simulink model "prototype_multiple_msg"  (R2021b)
settings: Solver=FixedStepDiscrete  StartTime=0.0  StopTime=Inf  FixedStep=1  RelTol=1e-3
settings Model: Creator=vgaggero  LastModifiedBy=grodriguez
settings SolverCC: AllowMultiTaskInputOutput=on  AutoInsertRateTranBlk=on  InsertRTBMode=Never (minimum delay)

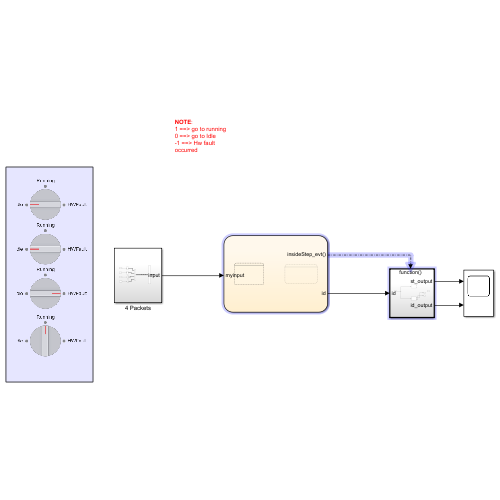
[thumbnail: Simulink's stored preview of the top-level diagram]
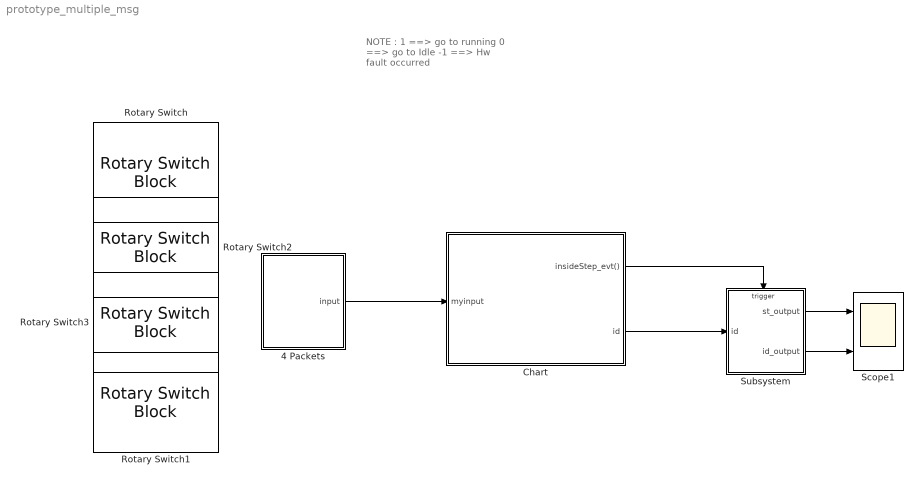
== system prototype_multiple_msg ==
  note: NOTE :
      | 1 ==> go to running
      | 0 ==> go to Idle
      | -1 ==> Hw fault occurred
  4 Packets : Subsystem
  Chart : Stateflow chart  TreatAsAtomicUnit=on
      settings: PortSchema="{\"entries\":[{\"content\":{\"sides\":[{\"content\":{\"connectorIds\":[\"In1\"]},\"type\":\"ConnectorPlacement.EquallySpacedRectSide\",\"uuid\":\"6cfd0d6c-bd6f-4458-8e18-10a89c7a7397\"},{\"content\":{\"connectorIds\":[\"Out2\",\"Out1\"],\"side\":\"RIGHT\"},\"type\":\"ConnectorPlacement.EquallySpacedRectSide\",\"uuid\":\"2cbad870-62d0-4bb8-9198-36e7d278500c\"},{\"content\":{\"connectorIds\":[],\"side\":\"TOP\"},\"type\":\"ConnectorPlacement.EquallySpacedRectSide\",\"uuid\":\"c9b4a32e-c2b5-43d7-b3cd-6996e0fae254\"}]},\"type\":\"ConnectorPlacement.EquallySpacedConnector\",\"uuid\":\"e32f82e2-d4b7-4dda-bf5a-9df2c9c9d870\"}],\"packageUris\":[\"http://schema.mathworks.com/mf0/Connector/R2020b\"],\"version\":\"1.0\"}"
  Rotary Switch{,1..3} (4 alike) : RotarySwitchBlock  LabelPosition=Hide
      settings: Values={{'Idle', 'Running', 'HWFault'}, [0 1 -1]}
  Scope1 : Scope  NumInputPorts=2
  Subsystem : Subsystem
  wires:
  Chart/2(insideStep_evt()) -> Subsystem/Trigger
  Chart/1(id) -> Subsystem/1(id)
  Subsystem/1(st_output) -> Scope1/1
  Subsystem/2(id_output) -> Scope1/2
  4 Packets/1(input) -> Chart/1(myinput)

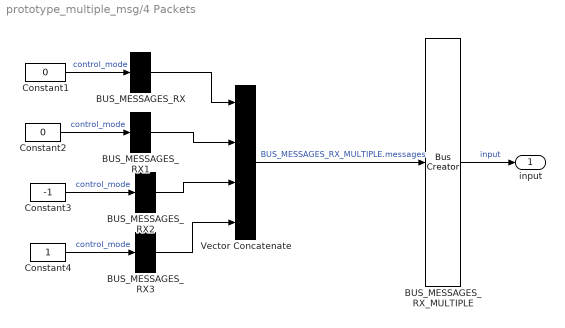
== system prototype_multiple_msg/4 Packets ==
  BUS_MESSAGES_RX{,1..3} (4 alike) : BusCreator  Inputs=1  OutDataTypeStr=Bus: BUS_MESSAGES_RX  NonVirtualBus=on
  BUS_MESSAGES_RX_MULTIPLE : BusCreator  Inputs=1  OutDataTypeStr=Bus: BUS_MESSAGES_RX_MULTIPLE  NonVirtualBus=on
  Constant1 : Constant  Value=0  OutDataTypeStr=int32
  Constant2 : Constant  Value=0  OutDataTypeStr=int32
  Constant3 : Constant  Value=-1  OutDataTypeStr=int32
  Constant4 : Constant  OutDataTypeStr=int32
  Vector Concatenate : Concatenate  NumInputs=4
  input : Outport
  wires:
  Constant2/1 -> BUS_MESSAGES_RX1/1  "control_mode"
  Constant1/1 -> BUS_MESSAGES_RX/1  "control_mode"
  Constant3/1 -> BUS_MESSAGES_RX2/1  "control_mode"
  BUS_MESSAGES_RX3/1 -> Vector Concatenate/4
  Constant4/1 -> BUS_MESSAGES_RX3/1  "control_mode"
  BUS_MESSAGES_RX/1 -> Vector Concatenate/1
  Vector Concatenate/1 -> BUS_MESSAGES_RX_MULTIPLE/1  "BUS_MESSAGES_RX_MULTIPLE.messages"
  BUS_MESSAGES_RX1/1 -> Vector Concatenate/2
  BUS_MESSAGES_RX2/1 -> Vector Concatenate/3
  BUS_MESSAGES_RX_MULTIPLE/1 -> input/1  "input"

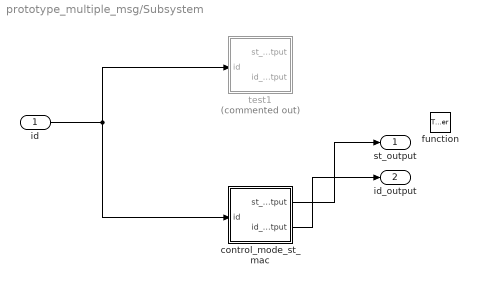
== system prototype_multiple_msg/Subsystem ==
  id : Inport
  function : TriggerPort  TriggerType=function-call  VariantControl=(inherit)
  control_mode_st_mac : Stateflow chart  TreatAsAtomicUnit=on
  test1 : Stateflow chart  Commented=on  TreatAsAtomicUnit=on
  st_output : Outport
  id_output : Outport  Port=2
  wires:
  id/1 -> control_mode_st_mac/1(id), test1/1(id)
  control_mode_st_mac/1(st_output) -> st_output/1
  control_mode_st_mac/2(id_output) -> id_output/1

== stateflow chart prototype_multiple_msg/Subsystem/control_mode_st_mac ==
  state Idle
    entry:
    id_output=id;
    st_output=0;
  state Running
    entry:
    id_output=id;
    st_output=10;
  state HwFault
    entry:
    id_output=id;
    st_output=20;
  (default) -> Idle
  Idle -> Running [order 1] : [id==1]
  HwFault -> Idle : [id==0]
  Idle -> HwFault [order 2] : [id==-1]
  Running -> HwFault : [id==-1]
  data: st_output output int32 size=1; id input int32 size=1; id_output output int32 size=1

== stateflow chart prototype_multiple_msg/Subsystem/test1 ==
  state Running
    entry:
    id_output=id;
    st_output=10;
  state HwFault
    entry:
    id_output=id;
    st_output=20;
  state HwFault1
    entry:
    id_output=id;
    st_output=30;
  state HwFault4
    entry:
    id_output=id;
    st_output=40;
  state HwFault3
    entry:
    id_output=id;
    st_output=50;
  state HwFault2
    entry:
    id_output=id;
    st_output=60;
  state Idle
    entry:
    id_output=id;
    st_output=0;
  (default) -> Idle
  Running -> HwFault : [id<5]
  Idle -> Running
  HwFault -> HwFault1
  HwFault1 -> HwFault4
  HwFault4 -> HwFault3
  HwFault3 -> HwFault2
  HwFault2 -> Idle
  data: st_output output int32 size=1; id input int32 size=1; id_output output int32 size=1

== stateflow chart prototype_multiple_msg/Chart ==
  state for_loop [parallel]
    settings: executionOrder=1
    state init
      entry:
    note: id=id+1;
    note: id=myinput.messages(index).control_mode;
    (default) -> init
    (junction 19) -> init
    init -> (junction 7) : {index=1}
    (junction 7) -> (junction 9) [order 1] : [index<5]
    (junction 9) -> (junction 11) : {id=myinput.messages(index).control_mode; send(insideStep_evt); }
    (junction 11) -> (junction 7) : {index = index + 1}
    (junction 7) -> (junction 19) [order 2]
  state my_state_machine [parallel] [commented out]
    state Home [commented out]
      entry:
      output=100;
      du:
      output=index;
    (default) -> Home [commented out]
    Home -> Home [commented out] : [insideStep_evt]{output=output+1;}
  data: myinput input Bus: BUS_MESSAGES_RX_MULTIPLE size=1; index local int32 size=1; id output int32 size=1 =int32(0)
  events: insideStep_evt output FUNCTION_CALL_EVENT
